simulink model "traffic_light_with_pedestrian"  (R2025a)
settings: Solver=FixedStepDiscrete  StartTime=0.0  StopTime=inf  FixedStep=1  RelTol=1e-3
settings Model: Creator=Issam  LastModifiedBy=Issam

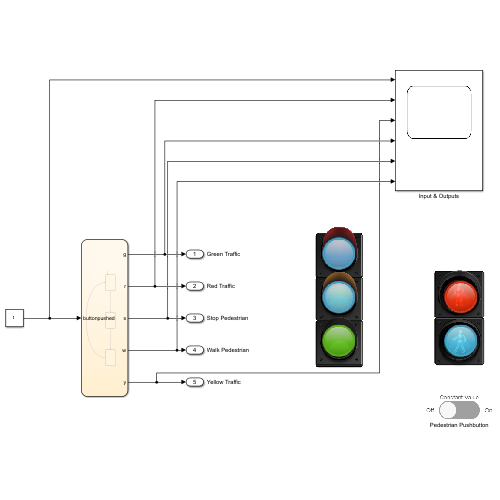
[thumbnail: Simulink's stored preview of the top-level diagram]
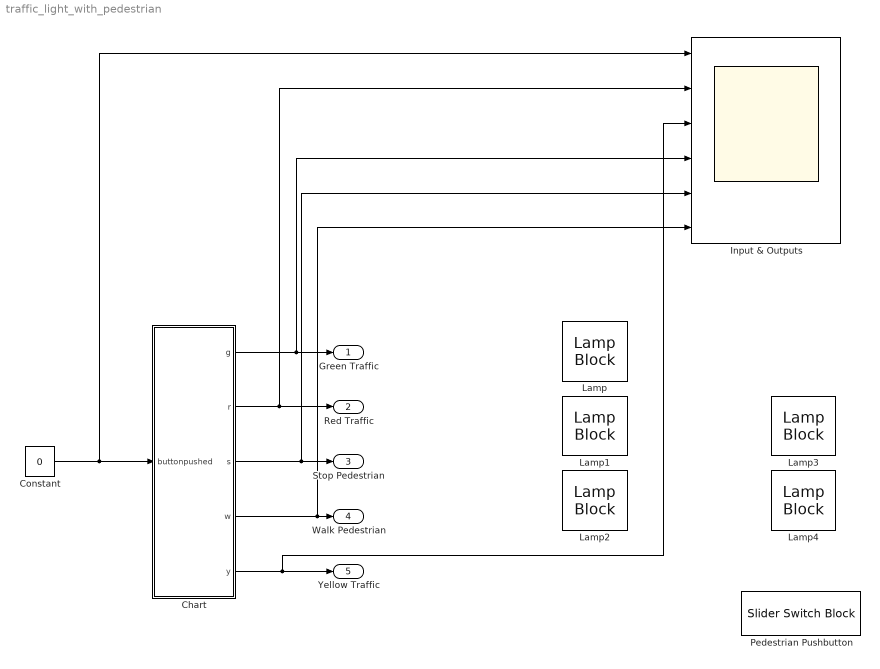
== system traffic_light_with_pedestrian ==
  Chart : Stateflow chart  TreatAsAtomicUnit=on
  Constant : Constant  Value=0
  Input & Outputs : Scope  NumInputPorts=6
      settings: ActiveDisplayString=5  ActiveDisplayYMinimum=-0.12499999999999997  ActiveDisplayYMaximum=1.125
  Lamp{,1..4} (5 alike) : LampBlock  LabelPosition=Hide  DefaultColor=[77.0, 190.0, 238.0]
  Pedestrian Pushbutton : SliderSwitchBlock
  Green Traffic : Outport
  Red Traffic : Outport  Port=2
  Stop Pedestrian : Outport  Port=3
  Walk Pedestrian : Outport  Port=4
  Yellow Traffic : Outport  Port=5
  wires:
  Chart/1(g) -> Input & Outputs/4, Green Traffic/1
  Chart/2(r) -> Input & Outputs/2, Red Traffic/1
  Chart/3(s) -> Input & Outputs/5, Stop Pedestrian/1
  Chart/4(w) -> Input & Outputs/6, Walk Pedestrian/1
  Chart/5(y) -> Input & Outputs/3, Yellow Traffic/1
  Constant/1 -> Input & Outputs/1, Chart/1(buttonpushed)

== stateflow chart traffic_light_with_pedestrian/Chart ==
  settings: sampleTime=0.2
  state trafficgo
    entry:
    r = 0;
    y = 0;
    g = 1;gog
    w = 0;
    s = 1;
  state trafficcaution
    entry:
    r = 0;
    y = 1;
    g = 0;
    w = 0;
    s = 0;
  state trafficstop
    entry:
    r = 1;
    y = 0;
    g = 0;
    w = 1;
    s = 0;
  (default) -> trafficgo
  trafficstop -> trafficgo : after(6,tick)
  trafficgo -> trafficcaution : [buttonpushed ==1]
  trafficcaution -> trafficstop : after(3,tick)
  data: buttonpushed input; g output; r output; s output; w output; y output; gog constant double
